simulink model "AGV_2021_a"  (R2021a)
settings: Solver=FixedStepAuto  StartTime=0.0  StopTime=20  MaxStep=0.001  RelTol=1e-6
PreLoadFcn:
  | % first load parameters
  | initializeQuadrotorModel;
undefined symbols (not defined in the file): ctrl, quadrotor, simPar
libraries: pid_lib x4, sharedtransform x1
settings Model: Creator=beniamino  LastModifiedBy=epast
settings SolverCC: ZeroCrossAlgorithm=Adaptive  AlgebraicLoopSolver=TrustRegion
settings DebuggingCC: IgnoredZcDiagnostic=none

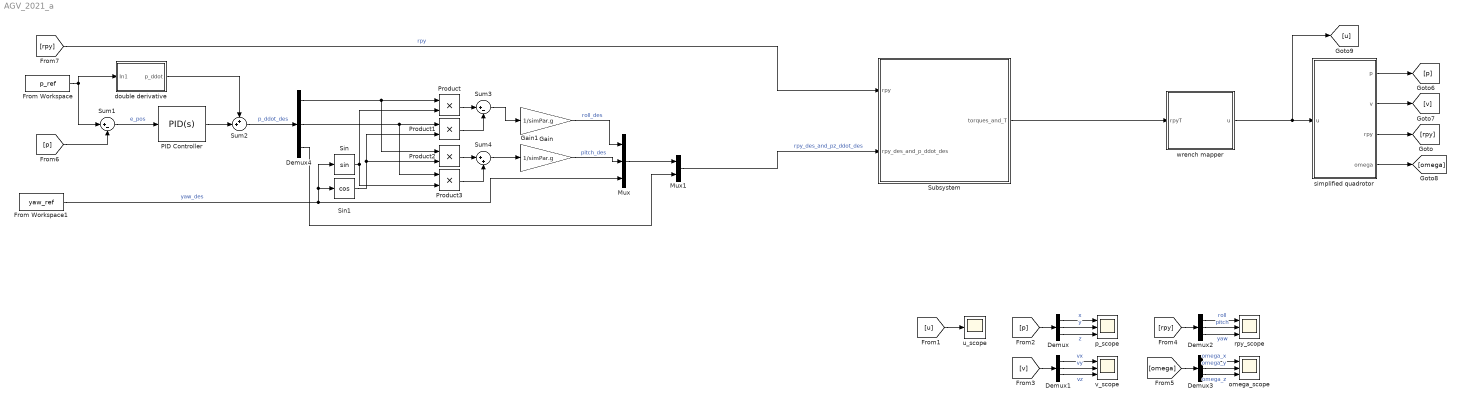
== system AGV_2021_a ==
  Demux{,1..4} (5 alike) : Demux  Outputs=3
  From Workspace : FromWorkspace  VariableName=p_ref
  From Workspace1 : FromWorkspace  VariableName=yaw_ref
  Gain : Gain  Gain=1/simPar.g
  Gain1 : Gain  Gain=1/simPar.g
  Mux : Mux  Inputs=3
  Mux1 : Mux  Inputs=2
  PID Controller : pid_lib/PID Controller  Controller=PID  Form=Parallel  TimeDomain=Continuous-time  UseExternalTs=off  SampleTime=-1  IntegratorMethod=Forward Euler  FilterMethod=Forward Euler  ControllerParametersSource=internal  P=15  I=0  D=6  UseFilter=on  N=100  TunerSelectOption=Transfer Function Based (PID Tuner App)  InitialConditionSource=internal  InitialConditionForIntegrator=0  InitialConditionForFilter=0  DifferentiatorICPrevScaledInput=0  ExternalReset=none  TrackingMode=off  Kt=1  LimitOutput=off  SatLimitsSource=internal  UpperSaturationLimit=inf  LowerSaturationLimit=-inf  LinearizeAsGain=on  AntiWindupMode=none  Kb=1  POutMin=[]  POutMax=[]  IOutMin=[]  IOutMax=[]  DOutMin=[]  DOutMax=[]  NOutMin=[]  NOutMax=[]  SumOutMin=[]  SumOutMax=[]  SaturationOutMin=[]  SaturationOutMax=[]  PParamMin=[]  PParamMax=[]  IParamMin=[]  IParamMax=[]  DParamMin=[]  DParamMax=[]  NParamMin=[]  NParamMax=[]  KbParamMin=[]  KbParamMax=[]  KtParamMin=[]  KtParamMax=[]  KbOutMin=[]  KbOutMax=[]  KtOutMin=[]  KtOutMax=[]  IntegratorOutMin=[]  IntegratorOutMax=[]  FilterOutMin=[]  FilterOutMax=[]  SumI1OutMin=[]  SumI1OutMax=[]  SumI2OutMin=[]  SumI2OutMax=[]  SumI3OutMin=[]  SumI3OutMax=[]  SumI4OutMin=[]  SumI4OutMax=[]  SumDOutMin=[]  SumDOutMax=[]  DifferentiatorOutMin=[]  DifferentiatorOutMax=[]  FilterDiffOutCoefMin=[]  FilterDiffOutCoefMax=[]  ReciprocalOutMin=[]  ReciprocalOutMax=[]  SumDenOutMin=[]  SumDenOutMax=[]  SumNumOutMin=[]  SumNumOutMax=[]  DivideOutMin=[]  DivideOutMax=[]  UdiffTsProdOutMin=[]  UdiffTsProdOutMax=[]  NTsProdOutMin=[]  NTsProdOutMax=[]  UintegralTsProdOutMin=[]  UintegralTsProdOutMax=[]  UngainTsProdOutMin=[]  UngainTsProdOutMax=[]  IntegratorContinuousStateAttributes=''  IntegratorStateMustResolveToSignalObject=off  IntegratorRTWStateStorageClass=Auto  FilterContinuousStateAttributes=''  FilterStateMustResolveToSignalObject=off  FilterRTWStateStorageClass=Auto  ParallelPVariant=InternalParameters  IdealPVariant=Disabled  IVariant=InternalParameters  DVariant=InternalParameters  IntegratorVariant=Continuous  SatVariant=Disabled  AWVariant=Passthrough  PCopyVariant=Disabled  TRVariant=Disabled  FdbkBlocksVariant=Forward  IdealPFdbkVariant=Disabled  SatFdbkVariant=Disabled  DerivativeFilterVariant=ContFilter  NVariant=InternalParameters  NCopyVariant=Disabled  FilterICVariant=InternalICsFilter  IntegratorICVariant=InternalICs  ExternalResetVariant=Disabled  TRSumVariant=Passthrough  SumFdbkVariant=Disabled  SumVariant=Sum_PID  TsampFilterVariant=InternalTs  TsampNgainVariant=Passthrough  TsampIntegralVariant=Passthrough  ExternalSaturationOutDataTypeStr=Inherit: Same as second input
  Product{,1..3} (4 alike) : Product
  Sin : Trigonometry
  Sin1 : Trigonometry  Operator=cos
  Subsystem : Subsystem
  Sum1 : Sum  Inputs=|+-
  Sum2 : Sum  Inputs=++|
  Sum3 : Sum  Inputs=|+-
  Sum4 : Sum  Inputs=|++
  double derivative : Subsystem
  omega_scope : Scope  NumInputPorts=3
  p_scope : Scope  NumInputPorts=3
  rpy_scope : Scope  NumInputPorts=3
  simplified quadrotor : Subsystem  mask(quadrotor model){F=quadrotor.mixer.F, M=quadrotor.mixer.M, mass=quadrotor.geometry.mass, gravity=simPar.g, inertia=quadrotor.geometry.I, maxRotorSpeed2=quadrotor.rotor.maxRotVelocity.^2, minRotorSpeed2=0, v_0=[0 0 0], omega_0=[0 0 0], ang_0=[0 0 0], p_0=[0 0 0]}
      mask prompts: F "F matrix"; M "M matrix"; mass "quadrotor mass"; inertia "inertia matrix"; maxRotorSpeed2 "Rotor max speed square"; minRotorSpeed2 "Rotor min speed square"; v_0 "initial linear velocity"; omega_0 "initial angular velocity"; ang_0 "initial angle"; p_0 "initial position"
      mask help: small angle simplified quadrotor model
      mask TypeOptions F: u2F/Gain
      mask TypeOptions M: u2M/Gain
      mask TypeOptions mass: mass/Value
      mask TypeOptions gravity: small angles rigid body dynamics/gravity/Value
      mask TypeOptions inertia: inertia/Value
      mask TypeOptions maxRotorSpeed2: saturate input/UpperLimit
      mask TypeOptions minRotorSpeed2: saturate input/LowerLimit
      mask TypeOptions v_0: small angles rigid body dynamics/ddp2dp/InitialCondition
      mask TypeOptions omega_0: small angles rigid body dynamics/domega2omega/InitialCondition
      mask TypeOptions ang_0: small angles rigid body dynamics/omega2ang/InitialCondition
      mask TypeOptions p_0: small angles rigid body dynamics/dp2p/InitialCondition
      mask DialogControl InitialConditionsGroupVar Prompt: Initial conditions
  u_scope : Scope
  v_scope : Scope  NumInputPorts=3
  wrench mapper : Subsystem  mask(wrench mapper){mapperMatrix=quadrotor.mixer.wrenchMapper}
      mask prompts: mapperMatrix "mapper matrix"
      mask help:
      | maps desired roll, pitch, yaw torque and total common thrust into the input vector u for a quadrotor.
      | input: [tau_roll, tau_pitch, tau_yaw, thrust]
      | input unit: [Nm, Nm, Nm, N]
      | output [u_1, u_2, u_3, u_3]
      | output unit: [rad^2/s^2]
      mask TypeOptions mapperMatrix: mapper/Gain
  wires:
  wrench mapper/1(u) -> [u], simplified quadrotor/1(u)
  simplified quadrotor/3(rpy) -> [rpy]
  simplified quadrotor/1(p) -> [p]
  simplified quadrotor/2(v) -> [v]
  simplified quadrotor/4(omega) -> [omega]
  [u] -> u_scope/1
  [p] -> Demux/1
  Demux/1 -> p_scope/1  "x"
  Demux/2 -> p_scope/2  "y"
  Demux/3 -> p_scope/3  "z"
  [v] -> Demux1/1
  Demux1/2 -> v_scope/2  "vy"
  Demux1/3 -> v_scope/3  "vz"
  Demux1/1 -> v_scope/1  "vx"
  [rpy] -> Demux2/1
  Demux2/2 -> rpy_scope/2  "pitch"
  Demux2/3 -> rpy_scope/3  "yaw"
  Demux2/1 -> rpy_scope/1  "roll"
  [omega] -> Demux3/1
  Demux3/2 -> omega_scope/2  "omega_y"
  Demux3/3 -> omega_scope/3  "omega_z"
  Demux3/1 -> omega_scope/1  "omega_x"
  From Workspace/1 -> double derivative/1(In1), Sum1/1
  [p] -> Sum1/2
  Sum1/1 -> PID Controller/1  "e_pos"
  PID Controller/1 -> Sum2/2
  Sum2/1 -> Demux4/1  "p_ddot_des"
  Demux4/2 -> Product3/1, Product1/1
  Demux4/3 -> Mux1/2
  Mux/1 -> Mux1/1
  From Workspace1/1 -> Mux/3, Sin1/1, Sin/1  "yaw_des"
  Gain/1 -> Mux/1  "roll_des"
  Gain1/1 -> Mux/2  "pitch_des"
  Sin/1 -> Product/2, Product3/2
  Sin1/1 -> Product2/2, Product1/2
  Product/1 -> Sum3/1
  Product1/1 -> Sum3/2
  Sum3/1 -> Gain/1
  Product3/1 -> Sum4/2
  Product2/1 -> Sum4/1
  Sum4/1 -> Gain1/1
  Demux4/1 -> Product2/1, Product/1
  [rpy] -> Subsystem/1(rpy)  "rpy"
  Mux1/1 -> Subsystem/2(rpy_des_and_p_ddot_des)  "rpy_des_and_pz_ddot_des"
  Subsystem/1(torques_and_T) -> wrench mapper/1(rpyT)
  double derivative/1(p_ddot) -> Sum2/1

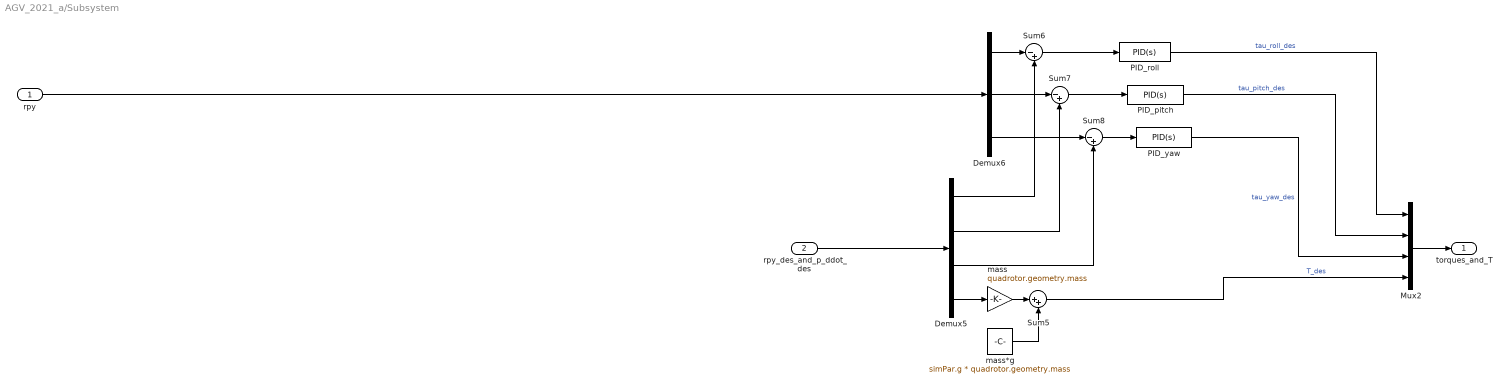
== system AGV_2021_a/Subsystem ==
  rpy : Inport
  rpy_des_and_p_ddot_des : Inport  Port=2
  Demux5 : Demux
  Demux6 : Demux  Outputs=3
  Mux2 : Mux
  PID_pitch : pid_lib/PID Controller  Controller=PID  Form=Parallel  TimeDomain=Continuous-time  UseExternalTs=off  SampleTime=-1  IntegratorMethod=Forward Euler  FilterMethod=Forward Euler  ControllerParametersSource=internal  P=ctrl.k_pitch_p  I=0  D=ctrl.k_pitch_d  UseFilter=on  N=ctrl.k_pitch_N  TunerSelectOption=Transfer Function Based (PID Tuner App)  InitialConditionSource=internal  InitialConditionForIntegrator=0  InitialConditionForFilter=0  DifferentiatorICPrevScaledInput=0  ExternalReset=none  TrackingMode=off  Kt=1  LimitOutput=off  SatLimitsSource=internal  UpperSaturationLimit=inf  LowerSaturationLimit=-inf  LinearizeAsGain=on  AntiWindupMode=none  Kb=1  POutMin=[]  POutMax=[]  IOutMin=[]  IOutMax=[]  DOutMin=[]  DOutMax=[]  NOutMin=[]  NOutMax=[]  SumOutMin=[]  SumOutMax=[]  SaturationOutMin=[]  SaturationOutMax=[]  PParamMin=[]  PParamMax=[]  IParamMin=[]  IParamMax=[]  DParamMin=[]  DParamMax=[]  NParamMin=[]  NParamMax=[]  KbParamMin=[]  KbParamMax=[]  KtParamMin=[]  KtParamMax=[]  KbOutMin=[]  KbOutMax=[]  KtOutMin=[]  KtOutMax=[]  IntegratorOutMin=[]  IntegratorOutMax=[]  FilterOutMin=[]  FilterOutMax=[]  SumI1OutMin=[]  SumI1OutMax=[]  SumI2OutMin=[]  SumI2OutMax=[]  SumI3OutMin=[]  SumI3OutMax=[]  SumI4OutMin=[]  SumI4OutMax=[]  SumDOutMin=[]  SumDOutMax=[]  DifferentiatorOutMin=[]  DifferentiatorOutMax=[]  FilterDiffOutCoefMin=[]  FilterDiffOutCoefMax=[]  ReciprocalOutMin=[]  ReciprocalOutMax=[]  SumDenOutMin=[]  SumDenOutMax=[]  SumNumOutMin=[]  SumNumOutMax=[]  DivideOutMin=[]  DivideOutMax=[]  UdiffTsProdOutMin=[]  UdiffTsProdOutMax=[]  NTsProdOutMin=[]  NTsProdOutMax=[]  UintegralTsProdOutMin=[]  UintegralTsProdOutMax=[]  UngainTsProdOutMin=[]  UngainTsProdOutMax=[]  IntegratorContinuousStateAttributes=''  IntegratorStateMustResolveToSignalObject=off  IntegratorRTWStateStorageClass=Auto  FilterContinuousStateAttributes=''  FilterStateMustResolveToSignalObject=off  FilterRTWStateStorageClass=Auto  ParallelPVariant=InternalParameters  IdealPVariant=Disabled  IVariant=InternalParameters  DVariant=InternalParameters  IntegratorVariant=Continuous  SatVariant=Disabled  AWVariant=Passthrough  PCopyVariant=Disabled  TRVariant=Disabled  FdbkBlocksVariant=Forward  IdealPFdbkVariant=Disabled  SatFdbkVariant=Disabled  DerivativeFilterVariant=ContFilter  NVariant=InternalParameters  NCopyVariant=Disabled  FilterICVariant=InternalICsFilter  IntegratorICVariant=InternalICs  ExternalResetVariant=Disabled  TRSumVariant=Passthrough  SumFdbkVariant=Disabled  SumVariant=Sum_PID  TsampFilterVariant=InternalTs  TsampNgainVariant=Passthrough  TsampIntegralVariant=Passthrough  ExternalSaturationOutDataTypeStr=Inherit: Same as second input
  PID_roll : pid_lib/PID Controller  Controller=PID  Form=Parallel  TimeDomain=Continuous-time  UseExternalTs=off  SampleTime=-1  IntegratorMethod=Forward Euler  FilterMethod=Forward Euler  ControllerParametersSource=internal  P=ctrl.k_roll_p  I=0  D=ctrl.k_roll_d  UseFilter=on  N=ctrl.k_roll_N  TunerSelectOption=Transfer Function Based (PID Tuner App)  InitialConditionSource=internal  InitialConditionForIntegrator=0  InitialConditionForFilter=0  DifferentiatorICPrevScaledInput=0  ExternalReset=none  TrackingMode=off  Kt=1  LimitOutput=off  SatLimitsSource=internal  UpperSaturationLimit=inf  LowerSaturationLimit=-inf  LinearizeAsGain=on  AntiWindupMode=none  Kb=1  POutMin=[]  POutMax=[]  IOutMin=[]  IOutMax=[]  DOutMin=[]  DOutMax=[]  NOutMin=[]  NOutMax=[]  SumOutMin=[]  SumOutMax=[]  SaturationOutMin=[]  SaturationOutMax=[]  PParamMin=[]  PParamMax=[]  IParamMin=[]  IParamMax=[]  DParamMin=[]  DParamMax=[]  NParamMin=[]  NParamMax=[]  KbParamMin=[]  KbParamMax=[]  KtParamMin=[]  KtParamMax=[]  KbOutMin=[]  KbOutMax=[]  KtOutMin=[]  KtOutMax=[]  IntegratorOutMin=[]  IntegratorOutMax=[]  FilterOutMin=[]  FilterOutMax=[]  SumI1OutMin=[]  SumI1OutMax=[]  SumI2OutMin=[]  SumI2OutMax=[]  SumI3OutMin=[]  SumI3OutMax=[]  SumI4OutMin=[]  SumI4OutMax=[]  SumDOutMin=[]  SumDOutMax=[]  DifferentiatorOutMin=[]  DifferentiatorOutMax=[]  FilterDiffOutCoefMin=[]  FilterDiffOutCoefMax=[]  ReciprocalOutMin=[]  ReciprocalOutMax=[]  SumDenOutMin=[]  SumDenOutMax=[]  SumNumOutMin=[]  SumNumOutMax=[]  DivideOutMin=[]  DivideOutMax=[]  UdiffTsProdOutMin=[]  UdiffTsProdOutMax=[]  NTsProdOutMin=[]  NTsProdOutMax=[]  UintegralTsProdOutMin=[]  UintegralTsProdOutMax=[]  UngainTsProdOutMin=[]  UngainTsProdOutMax=[]  IntegratorContinuousStateAttributes=''  IntegratorStateMustResolveToSignalObject=off  IntegratorRTWStateStorageClass=Auto  FilterContinuousStateAttributes=''  FilterStateMustResolveToSignalObject=off  FilterRTWStateStorageClass=Auto  ParallelPVariant=InternalParameters  IdealPVariant=Disabled  IVariant=InternalParameters  DVariant=InternalParameters  IntegratorVariant=Continuous  SatVariant=Disabled  AWVariant=Passthrough  PCopyVariant=Disabled  TRVariant=Disabled  FdbkBlocksVariant=Forward  IdealPFdbkVariant=Disabled  SatFdbkVariant=Disabled  DerivativeFilterVariant=ContFilter  NVariant=InternalParameters  NCopyVariant=Disabled  FilterICVariant=InternalICsFilter  IntegratorICVariant=InternalICs  ExternalResetVariant=Disabled  TRSumVariant=Passthrough  SumFdbkVariant=Disabled  SumVariant=Sum_PID  TsampFilterVariant=InternalTs  TsampNgainVariant=Passthrough  TsampIntegralVariant=Passthrough  ExternalSaturationOutDataTypeStr=Inherit: Same as second input
  PID_yaw : pid_lib/PID Controller  Controller=PID  Form=Parallel  TimeDomain=Continuous-time  UseExternalTs=off  SampleTime=-1  IntegratorMethod=Forward Euler  FilterMethod=Forward Euler  ControllerParametersSource=internal  P=ctrl.k_yaw_p  I=0  D=ctrl.k_yaw_d  UseFilter=on  N=ctrl.k_yaw_N  TunerSelectOption=Frequency Response Based  InitialConditionSource=internal  InitialConditionForIntegrator=0  InitialConditionForFilter=0  DifferentiatorICPrevScaledInput=0  ExternalReset=none  TrackingMode=off  Kt=1  LimitOutput=off  SatLimitsSource=internal  UpperSaturationLimit=inf  LowerSaturationLimit=-inf  LinearizeAsGain=on  AntiWindupMode=none  Kb=1  POutMin=[]  POutMax=[]  IOutMin=[]  IOutMax=[]  DOutMin=[]  DOutMax=[]  NOutMin=[]  NOutMax=[]  SumOutMin=[]  SumOutMax=[]  SaturationOutMin=[]  SaturationOutMax=[]  PParamMin=[]  PParamMax=[]  IParamMin=[]  IParamMax=[]  DParamMin=[]  DParamMax=[]  NParamMin=[]  NParamMax=[]  KbParamMin=[]  KbParamMax=[]  KtParamMin=[]  KtParamMax=[]  KbOutMin=[]  KbOutMax=[]  KtOutMin=[]  KtOutMax=[]  IntegratorOutMin=[]  IntegratorOutMax=[]  FilterOutMin=[]  FilterOutMax=[]  SumI1OutMin=[]  SumI1OutMax=[]  SumI2OutMin=[]  SumI2OutMax=[]  SumI3OutMin=[]  SumI3OutMax=[]  SumI4OutMin=[]  SumI4OutMax=[]  SumDOutMin=[]  SumDOutMax=[]  DifferentiatorOutMin=[]  DifferentiatorOutMax=[]  FilterDiffOutCoefMin=[]  FilterDiffOutCoefMax=[]  ReciprocalOutMin=[]  ReciprocalOutMax=[]  SumDenOutMin=[]  SumDenOutMax=[]  SumNumOutMin=[]  SumNumOutMax=[]  DivideOutMin=[]  DivideOutMax=[]  UdiffTsProdOutMin=[]  UdiffTsProdOutMax=[]  NTsProdOutMin=[]  NTsProdOutMax=[]  UintegralTsProdOutMin=[]  UintegralTsProdOutMax=[]  UngainTsProdOutMin=[]  UngainTsProdOutMax=[]  IntegratorContinuousStateAttributes=''  IntegratorStateMustResolveToSignalObject=off  IntegratorRTWStateStorageClass=Auto  FilterContinuousStateAttributes=''  FilterStateMustResolveToSignalObject=off  FilterRTWStateStorageClass=Auto  ParallelPVariant=InternalParameters  IdealPVariant=Disabled  IVariant=InternalParameters  DVariant=InternalParameters  IntegratorVariant=Continuous  SatVariant=Disabled  AWVariant=Passthrough  PCopyVariant=Disabled  TRVariant=Disabled  FdbkBlocksVariant=Forward  IdealPFdbkVariant=Disabled  SatFdbkVariant=Disabled  DerivativeFilterVariant=ContFilter  NVariant=InternalParameters  NCopyVariant=Disabled  FilterICVariant=InternalICsFilter  IntegratorICVariant=InternalICs  ExternalResetVariant=Disabled  TRSumVariant=Passthrough  SumFdbkVariant=Disabled  SumVariant=Sum_PID  TsampFilterVariant=InternalTs  TsampNgainVariant=Passthrough  TsampIntegralVariant=Passthrough  ExternalSaturationOutDataTypeStr=Inherit: Same as second input
  Sum5 : Sum  Inputs=|++
  Sum6 : Sum  Inputs=|-+
  Sum7 : Sum  Inputs=|-+
  Sum8 : Sum  Inputs=|-+
  mass : Gain  Gain=quadrotor.geometry.mass
  mass*g : Constant  Value=simPar.g * quadrotor.geometry.mass
  torques_and_T : Outport
  wires:
  PID_yaw/1 -> Mux2/3  "tau_yaw_des"
  Sum5/1 -> Mux2/4  "T_des"
  Mux2/1 -> torques_and_T/1
  rpy/1 -> Demux6/1
  mass*g/1 -> Sum5/2
  PID_roll/1 -> Mux2/1  "tau_roll_des"
  PID_pitch/1 -> Mux2/2  "tau_pitch_des"
  Demux5/4 -> mass/1
  rpy_des_and_p_ddot_des/1 -> Demux5/1
  mass/1 -> Sum5/1
  Demux6/1 -> Sum6/1
  Demux5/1 -> Sum6/2
  Demux6/2 -> Sum7/1
  Demux5/2 -> Sum7/2
  Demux6/3 -> Sum8/1
  Demux5/3 -> Sum8/2
  Sum6/1 -> PID_roll/1
  Sum7/1 -> PID_pitch/1
  Sum8/1 -> PID_yaw/1

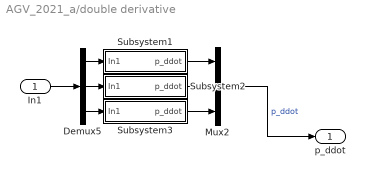
== system AGV_2021_a/double derivative ==
  In1 : Inport
  Demux5 : Demux  Outputs=3
  Mux2 : Mux  Inputs=3
  Subsystem1 : Subsystem
  Subsystem2 : Subsystem
  Subsystem3 : Subsystem
  p_ddot : Outport
  wires:
  Demux5/1 -> Subsystem1/1(In1)
  Demux5/2 -> Subsystem2/1(In1)
  Demux5/3 -> Subsystem3/1(In1)
  Subsystem2/1(p_ddot) -> Mux2/2
  Subsystem1/1(p_ddot) -> Mux2/1
  In1/1 -> Demux5/1
  Subsystem3/1(p_ddot) -> Mux2/3
  Mux2/1 -> p_ddot/1  "p_ddot"

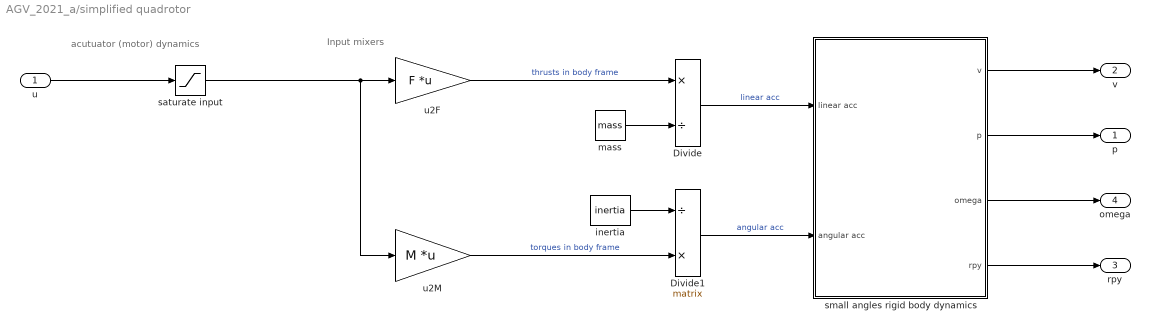
== system AGV_2021_a/simplified quadrotor ==
  note: Input mixers
  note: acutuator (motor) dynamics
  u : Inport
  Divide : Product  Inputs=*/
  Divide1 : Product  Inputs=/*  Multiplication=Matrix(*)
  inertia : Constant  Value=inertia
  mass : Constant  Value=mass
  saturate input : Saturate  UpperLimit=maxRotorSpeed2  LowerLimit=minRotorSpeed2
  small angles rigid body dynamics : Subsystem
  u2F : Gain  Gain=F  Multiplication=Matrix(K*u)
  u2M : Gain  Gain=M  Multiplication=Matrix(K*u)
  p : Outport  PortDimensions=3
  v : Outport  Port=2  PortDimensions=3
  rpy : Outport  Port=3  PortDimensions=3
  omega : Outport  Port=4  PortDimensions=3
  wires:
  small angles rigid body dynamics/4(rpy) -> rpy/1
  small angles rigid body dynamics/3(omega) -> omega/1
  small angles rigid body dynamics/2(p) -> p/1
  small angles rigid body dynamics/1(v) -> v/1
  Divide1/1 -> small angles rigid body dynamics/2(angular acc)  "angular acc"
  Divide/1 -> small angles rigid body dynamics/1(linear acc)  "linear acc"
  u/1 -> saturate input/1
  inertia/1 -> Divide1/1
  u2M/1 -> Divide1/2  "torques in body frame"
  u2F/1 -> Divide/1  "thrusts in body frame"
  mass/1 -> Divide/2
  saturate input/1 -> u2F/1, u2M/1

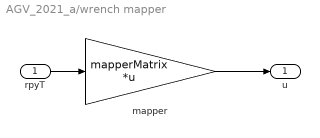
== system AGV_2021_a/wrench mapper ==
  rpyT : Inport
  mapper : Gain  Gain=mapperMatrix  Multiplication=Matrix(K*u)
  u : Outport
  wires:
  mapper/1 -> u/1
  rpyT/1 -> mapper/1

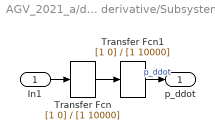
== system AGV_2021_a/double derivative/Subsystem1 ==
  In1 : Inport
  Transfer Fcn : TransferFcn  Numerator=[1 0]  Denominator=[1 10000]
  Transfer Fcn1 : TransferFcn  Numerator=[1 0]  Denominator=[1 10000]
  p_ddot : Outport
  wires:
  Transfer Fcn/1 -> Transfer Fcn1/1
  In1/1 -> Transfer Fcn/1
  Transfer Fcn1/1 -> p_ddot/1  "p_ddot"

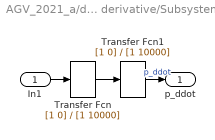
== system AGV_2021_a/double derivative/Subsystem2 ==
  In1 : Inport
  Transfer Fcn : TransferFcn  Numerator=[1 0]  Denominator=[1 10000]
  Transfer Fcn1 : TransferFcn  Numerator=[1 0]  Denominator=[1 10000]
  p_ddot : Outport
  wires:
  Transfer Fcn/1 -> Transfer Fcn1/1
  In1/1 -> Transfer Fcn/1
  Transfer Fcn1/1 -> p_ddot/1  "p_ddot"

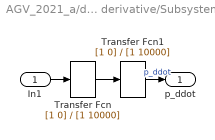
== system AGV_2021_a/double derivative/Subsystem3 ==
  In1 : Inport
  Transfer Fcn : TransferFcn  Numerator=[1 0]  Denominator=[1 10000]
  Transfer Fcn1 : TransferFcn  Numerator=[1 0]  Denominator=[1 10000]
  p_ddot : Outport
  wires:
  Transfer Fcn/1 -> Transfer Fcn1/1
  In1/1 -> Transfer Fcn/1
  Transfer Fcn1/1 -> p_ddot/1  "p_ddot"

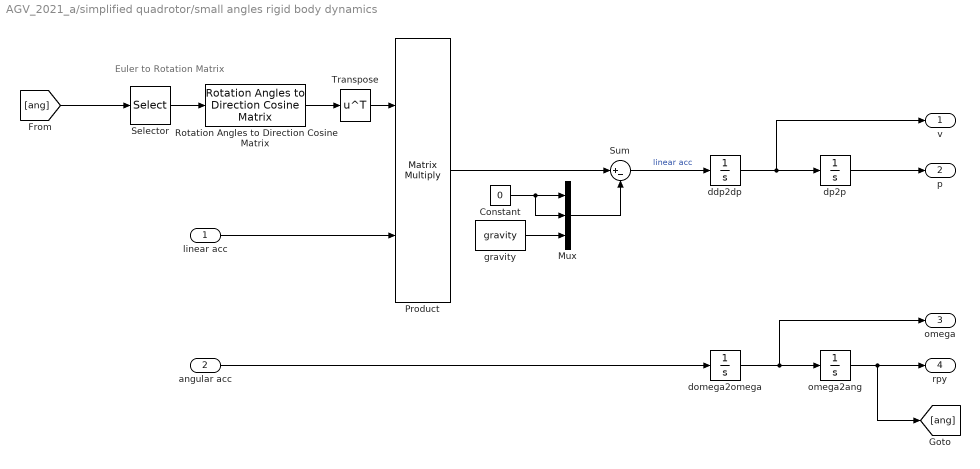
== system AGV_2021_a/simplified quadrotor/small angles rigid body dynamics ==
  note: Euler to Rotation Matrix
  linear acc : Inport
  angular acc : Inport  Port=2
  Constant : Constant  Value=0
  Mux : Mux  Inputs=3
  Product : Product  Multiplication=Matrix(*)
  Rotation Angles to Direction Cosine Matrix : sharedtransform/Rotation Angles to Direction Cosine Matrix  rotationOrder=ZYX  aMode=aMode
      settings: SourceProductBaseCode=AE,PW,DR,MT,UV,VE
  Selector : Selector  InputPortWidth=3  IndexOptions=Index vector (dialog)  Indices=[3 2 1]  OutputSizes=1
  Sum : Sum  Inputs=|+-
  Transpose : Math  Operator=transpose  SaturateOnIntegerOverflow=on
  ddp2dp : Integrator  InitialCondition=v_0  ContinuousStateAttributes='v'
  domega2omega : Integrator  InitialCondition=omega_0  ContinuousStateAttributes='omega'
  dp2p : Integrator  InitialCondition=p_0  ContinuousStateAttributes='position'
  gravity : Constant  Value=gravity
  omega2ang : Integrator  InitialCondition=ang_0  ContinuousStateAttributes='rpy'
  v : Outport
  p : Outport  Port=2
  omega : Outport  Port=3
  rpy : Outport  Port=4
  wires:
  Mux/1 -> Sum/2
  [ang] -> Selector/1
  angular acc/1 -> domega2omega/1
  gravity/1 -> Mux/3
  ddp2dp/1 -> dp2p/1, v/1
  linear acc/1 -> Product/2
  Transpose/1 -> Product/1
  Product/1 -> Sum/1
  domega2omega/1 -> omega2ang/1, omega/1
  dp2p/1 -> p/1
  Sum/1 -> ddp2dp/1  "linear acc"
  Constant/1 -> Mux/1, Mux/2
  Selector/1 -> Rotation Angles to Direction Cosine Matrix/1
  omega2ang/1 -> [ang], rpy/1
  Rotation Angles to Direction Cosine Matrix/1 -> Transpose/1
